simulink model "Control_Hinf_con_Perturbaciones"  (R2025b)
settings: Solver=ode45  StartTime=0.0  StopTime=12  RelTol=1e-3
settings Model: Creator=Carlo  LastModifiedBy=Carlo
settings DataIOCC: SaveState=on

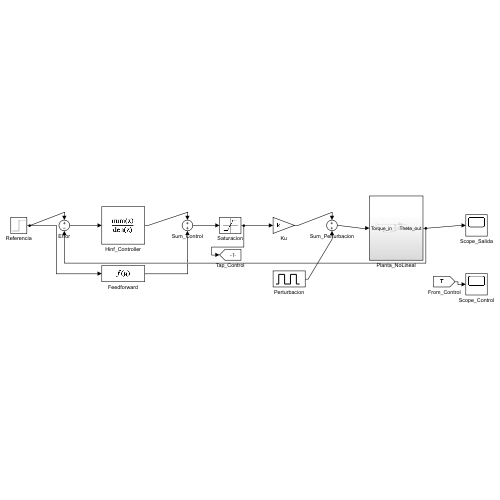
[thumbnail: Simulink's stored preview of the top-level diagram]
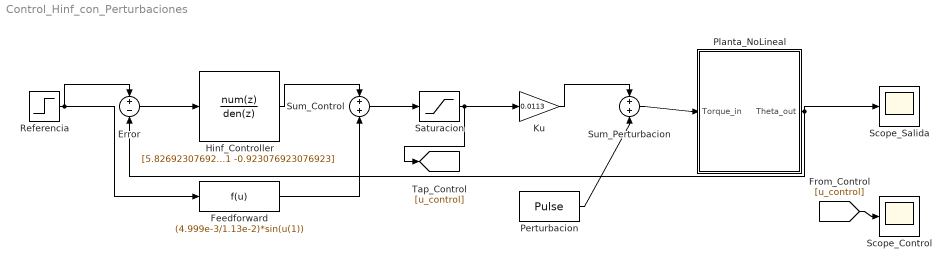
== system Control_Hinf_con_Perturbaciones ==
  Error : Sum  Inputs=+-
  Feedforward : Fcn  Expr=(4.999e-3/1.13e-2)*sin(u(1))
  Hinf_Controller : DiscreteTransferFcn  Numerator=[5.82692307692308 -5.71153846153846]  Denominator=[1 -0.923076923076923]  SampleTime=0.01
  Ku : Gain  Gain=0.0113
  Perturbacion : DiscretePulseGenerator  PulseType=Time based  Amplitude=0.002  Period=3  PulseWidth=20
  Planta_NoLineal : Subsystem
  Referencia : Step  Time=0  After=0.87266  SampleTime=0
  Saturacion : Saturate  UpperLimit=1  LowerLimit=-1
  Scope_Control : Scope
  Scope_Salida : Scope
      settings: ActiveDisplayYMinimum=0.86263840879166276  ActiveDisplayYMaximum=0.96285432087503464
  Sum_Control : Sum
  Sum_Perturbacion : Sum
  wires:
  Referencia/1 -> Error/1, Feedforward/1
  Error/1 -> Hinf_Controller/1
  Hinf_Controller/1 -> Sum_Control/1
  Sum_Control/1 -> Saturacion/1
  Saturacion/1 -> Ku/1, [u_control]
  Ku/1 -> Sum_Perturbacion/1
  Perturbacion/1 -> Sum_Perturbacion/2
  Sum_Perturbacion/1 -> Planta_NoLineal/1(Torque_in)
  Planta_NoLineal/1(Theta_out) -> Scope_Salida/1, Error/2
  Feedforward/1 -> Sum_Control/2
  [u_control] -> Scope_Control/1

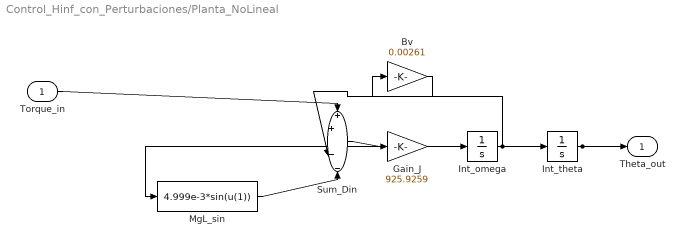
== system Control_Hinf_con_Perturbaciones/Planta_NoLineal ==
  Torque_in : Inport
  Bv : Gain  Gain=0.00261
  Gain_J : Gain  Gain=925.9259
  Int_omega : Integrator
  Int_theta : Integrator  InitialCondition=0.87266
  MgL_sin : Fcn  Expr=4.999e-3*sin(u(1))
  Sum_Din : Sum  Inputs=++--
  Theta_out : Outport
  wires:
  Torque_in/1 -> Sum_Din/1
  Sum_Din/1 -> Gain_J/1
  Gain_J/1 -> Int_omega/1
  Int_omega/1 -> Int_theta/1, Bv/1
  Int_theta/1 -> Theta_out/1, MgL_sin/1
  MgL_sin/1 -> Sum_Din/4
  Bv/1 -> Sum_Din/3
